simulink model "crazyflie"  (R2019b)
settings: Solver=FixedStepDiscrete  StartTime=0.0  StopTime=25  FixedStep=0.01  RelTol=1e-3
values from neighbouring files (symbols this model uses):
  r = r0    (= 1)    [get_LQR_gain.m]    (also in user_params.m = 0.98)
  Ts = 0.01    [params.m]    (also in user_params.m)
undefined symbols (not defined in the file or in its folder): DiscIntNeverNeededParam, K
settings Model: PauseTimes=7  Creator=Zrean  LastModifiedBy=parke
settings DataIOCC: ReturnWorkspaceOutputs=off
settings OptimizationCC: DefaultParameterBehavior=Inlined  UseDivisionForNetSlopeComputation=on  UseFloatMulNetSlope=on  UseSpecifiedMinMax=on  InlineInvariantSignals=on  PassReuseOutputArgsAs=Individual arguments  ZeroExternalMemoryAtStartup=off  ZeroInternalMemoryAtStartup=off  NoFixptDivByZeroProtection=on  EfficientFloat2IntCast=on  LifeSpan=1  EfficientTunableParamExpr=on
settings DebuggingCC: AlgebraicLoopMsg=error  ParameterTunabilityLossMsg=error  ArithmeticOperatorsInVariantConditions=warning
settings HardwareCC: ProdBitPerPointer=32  ProdBitPerSizeT=32  ProdBitPerPtrDiffT=32  ProdLargestAtomicInteger=Long  ProdLargestAtomicFloat=Double  ProdWordSize=32  ProdHWDeviceType=ARM Compatible->ARM Cortex
settings SFSimCC: SimUseLocalCustomCode=off  MATLABDynamicMemAlloc=off  CustomCodeUndefinedFunction=UseInterfaceOnly
settings RTWCC: SystemTargetFile=ert.tlc  GenCodeOnly=on  TemplateMakefile=ert_default_tmf  GenerateReport=on  RTWUseLocalCustomCode=off  BuildConfiguration=Faster Runs  IncludeHyperlinkInReport=on  LaunchReport=on  GenerateTraceInfo=on  GenerateTraceReport=on  GenerateTraceReportSl=on  GenerateTraceReportSf=on  GenerateTraceReportEml=on  GenerateCodeMetricsReport=on
settings CodeAppCC: ForceParamTrailComments=on  IgnoreCustomStorageClasses=off  OperatorAnnotations=on  SimulinkDataObjDesc=on  SFDataObjDesc=on  MATLABFcnDesc=on  InsertBlockDesc=on  StateflowObjectComments=on  MATLABSourceComments=on
settings ERTTargetCC: TargetLangStandard=C99 (ISO)  MultiwordLength=2048  CombineSignalStateStructs=on  SuppressErrorStatus=on  SupportAbsoluteTime=off  SupportNonFinite=off  SupportComplex=off  InlinedParameterPlacement=NonHierarchical  ERTCustomFileTemplate=crazyflie_wrapper.tlc  ERTFilePackagingFormat=CompactWithDataFile
settings SimscapeCC: SimscapeNormalizeSystem=off

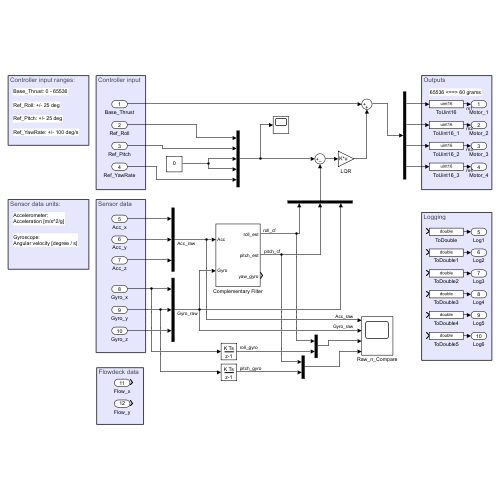
[thumbnail: Simulink's stored preview of the top-level diagram]
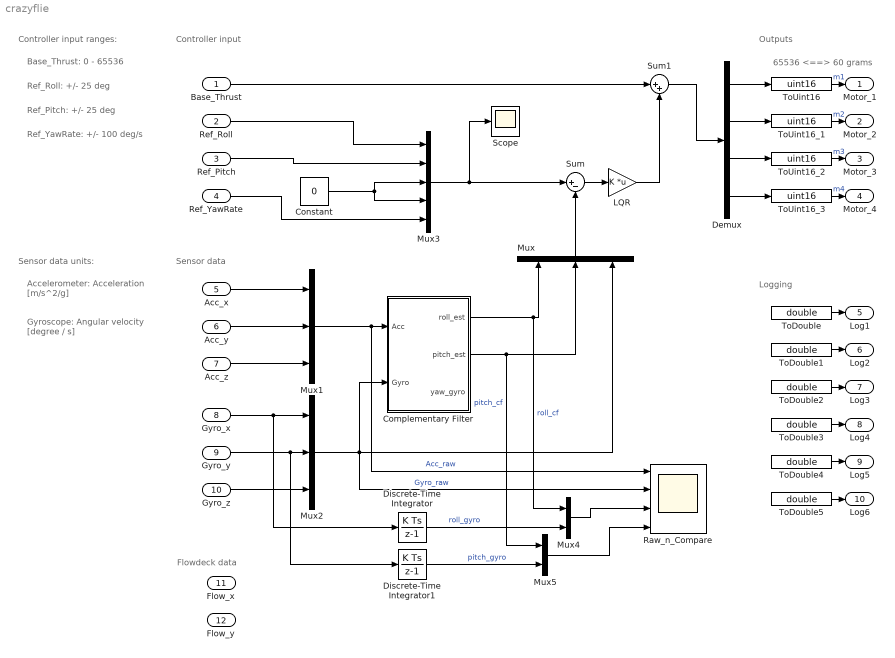
== system crazyflie ==
  note: 65536 <==> 60 grams
  note: Logging
  note: Outputs
  note: Sensor data
  note: Controller input
  note: Ref_Roll: +/- 25 deg
  note: Base_Thrust: 0 - 65536
  note: Ref_Pitch: +/- 25 deg
  note: Ref_YawRate: +/- 100 deg/s
  note: Controller input ranges:
  note: Gyroscope:
      | Angular velocity [degree / s]
  note: Accelerometer:
      | Acceleration [m/s^2/g]
  note: Sensor data units:
  note: Flowdeck data
  Base_Thrust : Inport  OutDataTypeStr=double
  Ref_Roll : Inport  Port=2  OutDataTypeStr=double
  Ref_Pitch : Inport  Port=3  OutDataTypeStr=double
  Ref_YawRate : Inport  Port=4  OutDataTypeStr=double
  Acc_x : Inport  Port=5  OutDataTypeStr=double  PortDimensions=1
  Acc_y : Inport  Port=6  OutDataTypeStr=double  PortDimensions=1
  Acc_z : Inport  Port=7  OutDataTypeStr=double  PortDimensions=1
  Gyro_x : Inport  Port=8  OutDataTypeStr=double  PortDimensions=1
  Gyro_y : Inport  Port=9  OutDataTypeStr=double  PortDimensions=1
  Gyro_z : Inport  Port=10  OutDataTypeStr=double  PortDimensions=1
  Flow_x : Inport  Port=11  OutDataTypeStr=int16  PortDimensions=1
  Flow_y : Inport  Port=12  OutDataTypeStr=int16  PortDimensions=1
  Complementary Filter : Subsystem
  Constant : Constant  Value=0
  Demux : Demux
  Discrete-Time Integrator : DiscreteIntegrator  gainval=1  SampleTime=Ts  ICPrevOutput=DiscIntNeverNeededParam  ICPrevScaledInput=DiscIntNeverNeededParam
  Discrete-Time Integrator1 : DiscreteIntegrator  gainval=1  SampleTime=Ts  ICPrevOutput=DiscIntNeverNeededParam  ICPrevScaledInput=DiscIntNeverNeededParam
  LQR : Gain  Gain=K  Multiplication=Matrix(K*u)
  Mux : Mux  Inputs=3
  Mux1 : Mux  Inputs=3
  Mux2 : Mux  Inputs=3
  Mux3 : Mux  Inputs=5
  Mux4 : Mux  Inputs=2
  Mux5 : Mux  Inputs=2
  Raw_n_Compare : Scope  NumInputPorts=4
  Scope : Scope
  Sum : Sum  Inputs=|+-
  Sum1 : Sum  Inputs=|++
  ToDouble{,1..5} (6 alike) : DataTypeConversion  OutDataTypeStr=double  SaturateOnIntegerOverflow=on
  ToUint16 : DataTypeConversion  OutDataTypeStr=uint16  SaturateOnIntegerOverflow=on
  ToUint16_1 : DataTypeConversion  OutDataTypeStr=uint16  SaturateOnIntegerOverflow=on
  ToUint16_2 : DataTypeConversion  OutDataTypeStr=uint16  SaturateOnIntegerOverflow=on
  ToUint16_3 : DataTypeConversion  OutDataTypeStr=uint16  SaturateOnIntegerOverflow=on
  Motor_1 : Outport  OutDataTypeStr=uint16  VectorParamsAs1DForOutWhenUnconnected=off  LockScale=on
  Motor_2 : Outport  Port=2  OutDataTypeStr=uint16  VectorParamsAs1DForOutWhenUnconnected=off  LockScale=on
  Motor_3 : Outport  Port=3  OutDataTypeStr=uint16  VectorParamsAs1DForOutWhenUnconnected=off  LockScale=on
  Motor_4 : Outport  Port=4  OutDataTypeStr=uint16  VectorParamsAs1DForOutWhenUnconnected=off  LockScale=on
  Log1 : Outport  Port=5  OutDataTypeStr=double  VectorParamsAs1DForOutWhenUnconnected=off
  Log2 : Outport  Port=6  OutDataTypeStr=double  VectorParamsAs1DForOutWhenUnconnected=off
  Log3 : Outport  Port=7  OutDataTypeStr=double  VectorParamsAs1DForOutWhenUnconnected=off
  Log4 : Outport  Port=8  OutDataTypeStr=double  VectorParamsAs1DForOutWhenUnconnected=off
  Log5 : Outport  Port=9  OutDataTypeStr=double  VectorParamsAs1DForOutWhenUnconnected=off
  Log6 : Outport  Port=10  OutDataTypeStr=double  VectorParamsAs1DForOutWhenUnconnected=off
  wires:
  ToUint16/1 -> Motor_1/1  "m1"
  ToUint16_1/1 -> Motor_2/1  "m2"
  ToUint16_2/1 -> Motor_3/1  "m3"
  ToUint16_3/1 -> Motor_4/1  "m4"
  ToDouble/1 -> Log1/1
  ToDouble1/1 -> Log2/1
  ToDouble2/1 -> Log3/1
  ToDouble3/1 -> Log4/1
  ToDouble4/1 -> Log5/1
  ToDouble5/1 -> Log6/1
  Acc_x/1 -> Mux1/1
  Acc_y/1 -> Mux1/2
  Acc_z/1 -> Mux1/3
  Discrete-Time Integrator/1 -> Mux4/2  "roll_gyro"
  Discrete-Time Integrator1/1 -> Mux5/2  "pitch_gyro"
  Mux4/1 -> Raw_n_Compare/3
  Mux5/1 -> Raw_n_Compare/4
  Gyro_x/1 -> Mux2/1, Discrete-Time Integrator/1
  Gyro_y/1 -> Discrete-Time Integrator1/1, Mux2/2
  Complementary Filter/1(roll_est) -> Mux4/1, Mux/1  "roll_cf"
  Complementary Filter/2(pitch_est) -> Mux/2, Mux5/1  "pitch_cf"
  Mux1/1 -> Complementary Filter/1(Acc), Raw_n_Compare/1  "Acc_raw"
  Mux2/1 -> Mux/3, Complementary Filter/2(Gyro), Raw_n_Compare/2  "Gyro_raw"
  Gyro_z/1 -> Mux2/3
  Mux/1 -> Sum/2
  Constant/1 -> Mux3/4, Mux3/3
  Mux3/1 -> Scope/1, Sum/1
  Ref_Roll/1 -> Mux3/1
  Ref_Pitch/1 -> Mux3/2
  Base_Thrust/1 -> Sum1/1
  Sum/1 -> LQR/1
  LQR/1 -> Sum1/2
  Demux/1 -> ToUint16/1
  Demux/2 -> ToUint16_1/1
  Demux/3 -> ToUint16_2/1
  Demux/4 -> ToUint16_3/1
  Sum1/1 -> Demux/1
  Ref_YawRate/1 -> Mux3/5

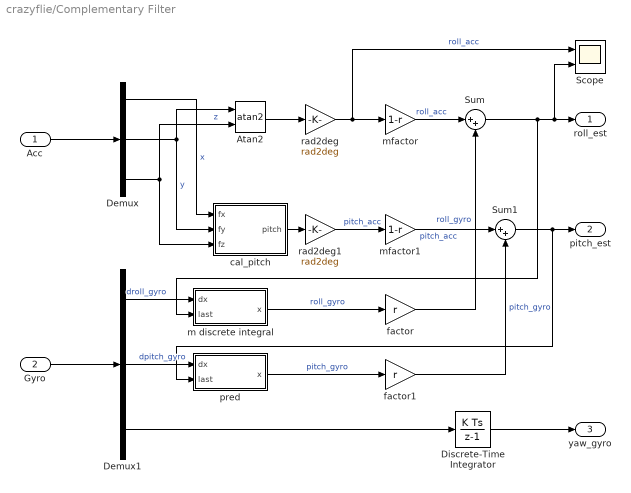
== system crazyflie/Complementary Filter ==
  Acc : Inport
  Gyro : Inport  Port=2
  Atan2 : Trigonometry  Operator=atan2
  Demux : Demux  Outputs=3
  Demux1 : Demux  Outputs=3
  Discrete-Time Integrator : DiscreteIntegrator  gainval=1  SampleTime=Ts  ICPrevOutput=DiscIntNeverNeededParam  ICPrevScaledInput=DiscIntNeverNeededParam
  Scope : Scope  NumInputPorts=2
  Sum : Sum  Inputs=|++
  Sum1 : Sum  Inputs=|++
  cal_pitch : MATLAB Function  TreatAsAtomicUnit=on
  factor : Gain  Gain=r
  factor1 : Gain  Gain=r
  m discrete integral : Subsystem
  mfactor : Gain  Gain=1-r
  mfactor1 : Gain  Gain=1-r
  pred : Subsystem
  rad2deg : Gain  Gain=rad2deg
  rad2deg1 : Gain  Gain=rad2deg
  roll_est : Outport  VectorParamsAs1DForOutWhenUnconnected=off
  pitch_est : Outport  Port=2  VectorParamsAs1DForOutWhenUnconnected=off
  yaw_gyro : Outport  Port=3  VectorParamsAs1DForOutWhenUnconnected=off
  wires:
  Acc/1 -> Demux/1
  Gyro/1 -> Demux1/1
  Demux/2 -> cal_pitch/2(fy), Atan2/1  "y"
  Demux/3 -> cal_pitch/3(fz), Atan2/2  "z"
  Atan2/1 -> rad2deg/1
  Sum/1 -> m discrete integral/2(last), Scope/2, roll_est/1
  rad2deg/1 -> Scope/1, mfactor/1  "roll_acc"
  mfactor/1 -> Sum/1  "roll_acc"
  factor/1 -> Sum/2  "roll_gyro"
  Demux1/1 -> m discrete integral/1(dx)  "droll_gyro"
  m discrete integral/1(x) -> factor/1  "roll_gyro"
  Demux1/2 -> pred/1(dx)  "dpitch_gyro"
  pred/1(x) -> factor1/1  "pitch_gyro"
  Demux/1 -> cal_pitch/1(fx)  "x"
  Demux1/3 -> Discrete-Time Integrator/1
  Discrete-Time Integrator/1 -> yaw_gyro/1
  cal_pitch/1(pitch) -> rad2deg1/1
  rad2deg1/1 -> mfactor1/1  "pitch_acc"
  Sum1/1 -> pitch_est/1, pred/2(last)
  mfactor1/1 -> Sum1/1  "pitch_acc"
  factor1/1 -> Sum1/2  "pitch_gyro"

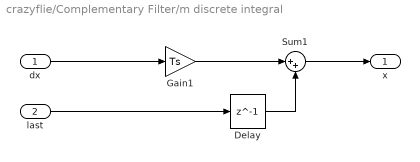
== system crazyflie/Complementary Filter/m discrete integral ==
  dx : Inport
  last : Inport  Port=2
  Delay : Delay  DelayLength=1  InitialCondition=0  SampleTime=Ts
  Gain1 : Gain  Gain=Ts
  Sum1 : Sum  Inputs=|++
  x : Outport  VectorParamsAs1DForOutWhenUnconnected=off
  wires:
  dx/1 -> Gain1/1
  Delay/1 -> Sum1/2
  last/1 -> Delay/1
  Sum1/1 -> x/1
  Gain1/1 -> Sum1/1

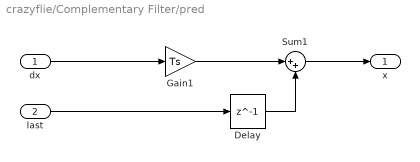
== system crazyflie/Complementary Filter/pred ==
  dx : Inport
  last : Inport  Port=2
  Delay : Delay  DelayLength=1  InitialCondition=0  SampleTime=Ts
  Gain1 : Gain  Gain=Ts
  Sum1 : Sum  Inputs=|++
  x : Outport  VectorParamsAs1DForOutWhenUnconnected=off
  wires:
  dx/1 -> Gain1/1
  Delay/1 -> Sum1/2
  last/1 -> Delay/1
  Sum1/1 -> x/1
  Gain1/1 -> Sum1/1

== matlab function crazyflie/Complementary Filter/cal_pitch ==
  data: fx input; pitch output; fy input; fz input
function pitch = fcn(fx, fy, fz)

pitch = atan2(-fx,norm([fy,fz]));
